simulink model "control"  (R2017b)
settings: Solver=VariableStepAuto  StartTime=0.0  StopTime=inf  RelTol=1e-3
values from neighbouring files (symbols this model uses):
  k = lqrd(A,B,Q,R,T)    [DIPV_LQR_gain_calculation.m]    (also in LQR_gain_calculation.m)
settings Model: Creator=lenovo  LastModifiedBy=lenovo

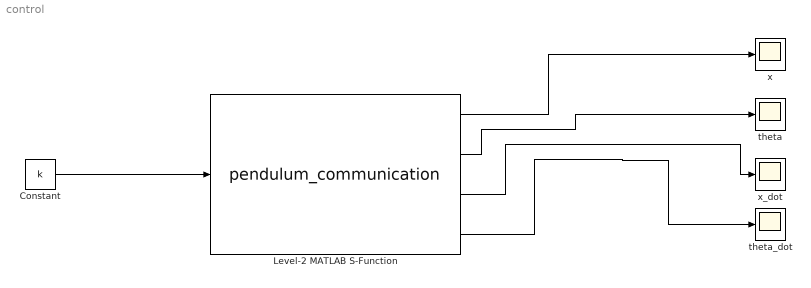
== system control ==
  Constant : Constant  Value=k  OutDataTypeStr=single  SampleTime=0.1
  Level-2 MATLAB S-Function : M-S-Function  FunctionName=pendulum_communication  Parameters=3 0.1
  theta : Scope
  theta_dot : Scope
  x : Scope
  x_dot : Scope
  wires:
  Level-2 MATLAB S-Function/1 -> x/1
  Level-2 MATLAB S-Function/2 -> theta/1
  Level-2 MATLAB S-Function/3 -> x_dot/1
  Level-2 MATLAB S-Function/4 -> theta_dot/1
  Constant/1 -> Level-2 MATLAB S-Function/1
